simulink model "LabAstationary"  (R2019a)
settings: Solver=ode5  StartTime=0.0  StopTime=500  RelTol=1e-3  EnableMultiTasking=on
values from neighbouring files (symbols this model uses):
  A = 33    [doubletank.m]    (also in fcn.m; jacobianA.m; kalman_dynamic.m; kalman_dynamic_EKF.m)
  a = 0.16    [doubletank.m]    (also in fcn.m; jacobianA.m; kalman_dynamic.m; kalman_dynamic_EKF.m)
  Amat = [ -(a*sqrt(2*g))/(2*A*sqrt(h10)) 0 ... (first row only)    [fcn.m]    (also in jacobianA.m = [df1dh1, df1dh2; df2dh1, df2dh2]; kalman_dynamic.m; kalman_dynamic_EKF.m; kalman_f_stationary.m)
  Bmat = [  (f_u - f_former)/(u - u_former); 0]    [fcn.m]    (also in kalman_dynamic.m = [6.22/A; 0]; kalman_dynamic_EKF.m = [6.22/A; 0]; kalman_f_stationary.m = [6.22/A; 0])
  Cmat = [0,1]    [fcn.m]    (also in kalman_dynamic.m = [0 1]; kalman_dynamic_EKF.m = [0 1]; kalman_f_stationary.m = [0 1])
  K = 5    [doubletank.m]    (also in fcn.m; kalman_dynamic.m; kalman_dynamic_EKF.m; kalman_f_stationary.m)
  u0 = 1.7    [fcn.m]    (also in kalman_dynamic.m; kalman_dynamic_EKF.m; kalman_f_stationary.m)
libraries: R7014E_lib x1
settings Model: Creator=wolfgang  LastModifiedBy=marbla-6
settings Model: ModifiedHistory=|
  | Created an adjusted empty Simulink diagram for the lab assignments
  | in the course R0002E
settings DataIOCC: SaveFormat=Array  SignalLoggingSaveFormat=ModelDataLogs  SaveOutput=off  SignalLogging=off  DSMLogging=off  SaveTime=off  ReturnWorkspaceOutputs=off
settings OptimizationCC: ExpressionDepthLimit=2147483647  LifeSpan=inf
settings DebuggingCC: UnderspecifiedInitializationDetection=Classic  MergeDetectMultiDrivingBlocksExec=none  SolverPrmCheckMsg=warning  FcnCallInpInsideContextMsg=warning  StateNameClashWarn=warning  SFUnexpectedBacktrackingDiag=warning  SFNoUnconditionalDefaultTransitionDiag=warning  SFExecutionAtInitializationDiag=none  ArithmeticOperatorsInVariantConditions=warning
settings HardwareCC: ProdBitPerPointer=32  ProdBitPerSizeT=32  ProdBitPerPtrDiffT=32  ProdLargestAtomicFloat=None  ProdIntDivRoundTo=Undefined  ProdEndianess=Unspecified  ProdWordSize=32  ProdHWDeviceType=32-bit Generic
settings ModelReferenceCC: PropagateSignalLabelsOutOfModel=off
settings SFSimCC: SimUseLocalCustomCode=off
settings RTWCC: RTWUseLocalCustomCode=off
settings CodeAppCC: StateflowObjectComments=on
settings GRTTargetCC: TargetLangStandard=C89/C90 (ANSI)  GeneratePreprocessorConditionals=Disable all
settings ConfigComp: CovMetricSettings=dw  CovHtmlReporting=on  CovSaveCumulativeToWorkspaceVar=on  CovSaveSingleToWorkspaceVar=on  CovExternalEMLEnable=off  CovSFcnEnable=off

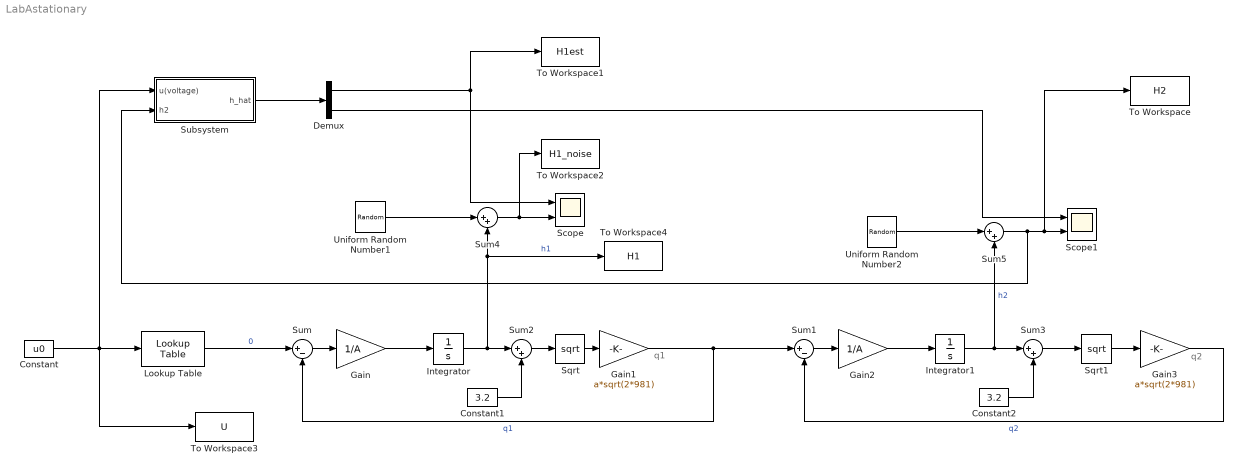
== system LabAstationary ==
  note: q1
  note: q2
  Constant : Constant  Value=u0  SampleTime=Inf
  Constant1 : Constant  Value=3.2
  Constant2 : Constant  Value=3.2
  Demux : Demux  Outputs=2
  Gain : Gain  Gain=1/A
  Gain1 : Gain  Gain=a*sqrt(2*981)
  Gain2 : Gain  Gain=1/A
  Gain3 : Gain  Gain=a*sqrt(2*981)
  Integrator : Integrator  LimitOutput=on  UpperSaturationLimit=15.5  LowerSaturationLimit=0
  Integrator1 : Integrator  LimitOutput=on  UpperSaturationLimit=15.5  LowerSaturationLimit=0
  Lookup Table : R7014E_lib/Lookup Table  x=[0.5,1,1.5,2,2.5,3,3.5,5,8,10]  y=[16.47,20.75,24.52,27.63,30.06,32.49,34.8,40.28,48.24,52.43]
  Scope : Scope  NumInputPorts=2
  Scope1 : Scope  NumInputPorts=2
  Sqrt : Sqrt  SaturateOnIntegerOverflow=on
  Sqrt1 : Sqrt  SaturateOnIntegerOverflow=on
  Subsystem : Subsystem
  Sum : Sum  Inputs=|+-
  Sum1 : Sum  Inputs=|+-
  Sum{2..5} (4 alike) : Sum  Inputs=|++
  To Workspace : ToWorkspace  VariableName=H2  SaveFormat=Timeseries  SampleTime=-1
  To Workspace1 : ToWorkspace  VariableName=H1est  SaveFormat=Timeseries  SampleTime=-1
  To Workspace2 : ToWorkspace  VariableName=H1_noise  SaveFormat=Timeseries  SampleTime=-1
  To Workspace3 : ToWorkspace  VariableName=U  SaveFormat=Timeseries  SampleTime=-1
  To Workspace4 : ToWorkspace  VariableName=H1  SaveFormat=Timeseries  SampleTime=-1
  Uniform Random Number1 : UniformRandomNumber  Minimum=-0.1  Maximum=0.1  SampleTime=0.1
  Uniform Random Number2 : UniformRandomNumber  Minimum=-0.1  Maximum=0.1  SampleTime=0.1
  wires:
  Sum/1 -> Gain/1
  Gain/1 -> Integrator/1
  Integrator/1 -> Sum2/1, To Workspace4/1, Sum4/2  "h1"
  Sqrt/1 -> Gain1/1
  Gain1/1 -> Sum1/1, Sum/2  "q1"
  Gain3/1 -> Sum1/2  "q2"
  Gain2/1 -> Integrator1/1
  Sqrt1/1 -> Gain3/1
  Sum1/1 -> Gain2/1
  Lookup Table/1 -> Sum/1  "0"
  Constant/1 -> To Workspace3/1, Lookup Table/1, Subsystem/1(u(voltage))
  Sum2/1 -> Sqrt/1
  Constant1/1 -> Sum2/2
  Constant2/1 -> Sum3/2
  Sum3/1 -> Sqrt1/1
  Uniform Random Number1/1 -> Sum4/1
  Integrator1/1 -> Sum3/1, Sum5/2  "h2"
  Uniform Random Number2/1 -> Sum5/1
  Subsystem/1(h_hat) -> Demux/1
  Sum5/1 -> Subsystem/2(h2), To Workspace/1, Scope1/2
  Demux/1 -> To Workspace1/1, Scope/1
  Demux/2 -> Scope1/1
  Sum4/1 -> Scope/2, To Workspace2/1

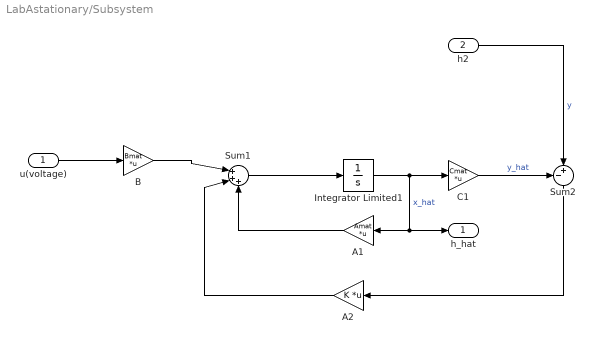
== system LabAstationary/Subsystem ==
  u(voltage) : Inport
  h2 : Inport  Port=2
  A1 : Gain  Gain=Amat  Multiplication=Matrix(K*u) (u vector)
  A2 : Gain  Gain=K  Multiplication=Matrix(K*u) (u vector)
  B : Gain  Gain=Bmat  Multiplication=Matrix(K*u) (u vector)
  C1 : Gain  Gain=Cmat  Multiplication=Matrix(K*u) (u vector)
  Integrator Limited1 : Integrator  LimitOutput=on  UpperSaturationLimit=15.5  LowerSaturationLimit=0
  Sum1 : Sum  Inputs=|+++
  Sum2 : Sum  Inputs=-+|
  h_hat : Outport
  wires:
  B/1 -> Sum1/1
  Integrator Limited1/1 -> h_hat/1, A1/1, C1/1  "x_hat"
  Sum1/1 -> Integrator Limited1/1
  A1/1 -> Sum1/3
  C1/1 -> Sum2/1  "y_hat"
  A2/1 -> Sum1/2
  Sum2/1 -> A2/1
  u(voltage)/1 -> B/1
  h2/1 -> Sum2/2  "y"
